simulink model "program_nova_torque_vectoring_001_2015b"  (R2016a)
settings: Solver=FixedStepAuto  StartTime=0.0  StopTime=10.0  RelTol=1e-3
PreLoadFcn:
  | dataCar
  | load_vars
  | readFuzzyFile
  | structAero
  | structEstimPar
  | structSensors
  | structSettings
PostLoadFcn:
  | , if any(exist('dsrtsu_mdlpostloadfcn', 'file') == [2, 3, 6]), try dsrtsu_mdlpostloadfcn('Execute', bdroot); catch fprintf('Error in PostLoadFcn (dsrtsu_mdlpostloadfcn) for model "%s":\n %s\n', bdroot, lasterr); end, end,
InitFcn:
  | dataCar
  | load_vars
  | readFuzzyFile
  | structAero
  | structEstimPar
  | structSensors
  | structSettings
StartFcn:
  | dataCar
  | load_vars
  | readFuzzyFile
  | structAero
  | structEstimPar
  | structSensors
  | structSettings
values from neighbouring files (symbols this model uses):
  Throttle2_offset = 500    [load_vars.m]
  Throttle_limits = [0.15, 0.90, 0.16, 0.92]    [load_vars.m]
libraries: rtican x42, hdlsllib x32, simulink x3, fuzblock x1
(part 11 of 11)

== matlab function program_nova_torque_vectoring_001_2015b/Processor/Vehicle Estimated Parameters/Fy Estimator  ==
  data: sensors input; Fyi output; settings input; Fzi input; Fxi input; car parameter
function Fyi = Fy_Estimator(sensors, settings, Fzi, Fxi, car)

Fyi=[0;0;0;0];
persistent yawRatePrev; if isempty(yawRatePrev); yawRatePrev = sensors.yawRate; end
persistent M_Fx; if isempty(M_Fx); M_Fx = 0; end
persistent M_Fy; if isempty(M_Fy); M_Fy = 0; end
persistent FyRear; if isempty(FyRear); FyRear = 0; end
persistent FzRatioFront; if isempty(FzRatioFront);FzRatioFront = 0; end
persistent FzRatioRear; if isempty(FzRatioRear); FzRatioRear = 0; end
persistent FyFront; if isempty(FyFront); FyFront = 0; end
persistent Fy_FL; if isempty(Fy_FL); Fy_FL = 0; end

scaleFactorFy = 0.7;

yawAcc = (sensors.yawRate - yawRatePrev) * car.fECU;

wheelAngle = (sensors.wheelAngles(1)+sensors.wheelAngles(2))/2;

%Calculate contributions to the moment from lateral forces through the
%total yaw moment and moment of the longitudinal forces.
M_YawTot = car.yawInertia*yawAcc;
M_Fx = (car.tw/2)*cos(wheelAngle)*(Fxi(1)-Fxi(2))...
    +car.lf*sin(wheelAngle)*(Fxi(1)+Fxi(2))...
    +(car.tw/2)*(Fxi(3)-Fxi(4));
M_Fy = M_YawTot - M_Fx;

%Distribution of lateral force on front and rear axle
%NOTE %sin(steerinAngle) deel wordt momenteel verwaarloosd
%     %--> FyFR - FyFL =~ 0
Fy = car.mass*sensors.ay;
FyRear = (cos(wheelAngle)*car.lf*Fy - M_Fy)/...
    (cos(wheelAngle)*car.lf+car.lr);
FyFront = Fy - FyRear;

%Distribution of lateral force on left and right tire by using the normal
%force distribution.

%Use of a scale factor 

FzRatioFront = [Fzi(1); Fzi(2)]./sum(Fzi(1:2));
FzRatioRear = [Fzi(3); Fzi(4)]./sum(Fzi(3:4));



FyFrontDiff = (FzRatioFront(1) - FzRatioFront(2))*scaleFactorFy/2;
Fy_FL = FyFront/2 + FyFrontDiff* FyFront;
Fy_FR = FyFront/2 - FyFrontDiff* FyFront;
FyRearDiff = (FzRatioRear(1) - FzRatioRear(2))*scaleFactorFy/2;
Fy_RL = FyRear/2 + FyRearDiff* FyRear;
Fy_RR = FyRear/2 - FyRearDiff* FyRear;
    
Fyi=[Fy_FL;Fy_FR;Fy_RL;Fy_RR];

yawRatePrev=sensors.yawRate;

== matlab function program_nova_torque_vectoring_001_2015b/Processor/Vehicle Estimated Parameters/Fz Estimator  ==
  data: sensors input; Fzi output; settings input; v input; car parameter; aero input
function Fzi = Fz_Estimator(sensors, settings, v,car, aero)
if isempty(v); v =0;end
%Dynamical loads 
%Without taking suspension into account


FFA = car.g*car.mass*car.lr/car.wb - (car.h/car.wb)*(car.mass*sensors.ax) - aero.FD*((car.h+aero.lever_FD(2))/car.wb) - aero.FL*((car.lr-aero.lever_FL(1))/car.wb); %dyn load Front Axle
FRA = car.g*car.mass*car.lf/car.wb + (car.h/car.wb)*(car.mass*sensors.ax) + aero.FD*((car.h+aero.lever_FD(2))/car.wb) - aero.FL*((car.lf+aero.lever_FL(1))/car.wb); %dyn load Rear Axle


FFL = FFA/2 - (car.h/(2*car.tw))*(car.mass*sensors.ay);
FFR = FFA/2 + (car.h/(2*car.tw))*(car.mass*sensors.ay);
FRL = FRA/2 - (car.h/(2*car.tw))*(car.mass*sensors.ay);
FRR = FRA/2 + (car.h/(2*car.tw))*(car.mass*sensors.ay);


Fzi = [FFL;FFR;FRL;FRR];

== matlab function program_nova_torque_vectoring_001_2015b/Processor/Vehicle Estimated Parameters/Mu&Slip Estimator ==
  data: sensors input; mu output; settings input; slip output; v input; car parameter
function [mu,slip]= mu_slip(sensors, settings,v,car)
if isempty(v); v =0;end
yawRate = [0;0;sensors.yawRate];
dist = [car.lf car.lf -car.lr -car.lr;
    car.tw/2 -car.tw/2 car.tw/2 -car.tw/2;
    0 0 0 0];
wheelAngle = (sensors.wheelAngles(1)+sensors.wheelAngles(2))/2;

mu=[car.mu;car.mu;car.mu;car.mu];

omegaR = sensors.wheelspeed*car.tireRadius;
vWheel=zeros(4,1);
vWheel_m=zeros(3,4);

for i=1:4;
    v_sleep=cross(yawRate,dist(:,i));
    vWheel_m(:,i) = [v;0;0] + v_sleep;
    vWheel(i,1) = sqrt(vWheel_m(1,i)^2+vWheel_m(2,i)^2);
end

%state.slipRatio = (sensor.omegaiWheel * car.wheelRadius - wvi)./max((sensor.omegaiWheel * car.wheelRadius),1);

if sensors.ax > 0
    slip = (omegaR - vWheel)./omegaR;
elseif sensors.ax < 0
    slip = (omegaR - vWheel)./vWheel;
else
    slip = [0;0;0;0];
end
end

== matlab function program_nova_torque_vectoring_001_2015b/Processor/Vehicle Estimated Parameters/Velocity Estimator/Fuzzy Velocity/FuzzyVelicityGenerator ==
  data: k1 input; vFuzzy output; k2 input; k3 input; k4 input; k5 input; sensors input; settings input; car parameter
function vFuzzy = fuzzyVelocityGenerator(k1,k2,k3,k4,k5,sensors,settings,car)

persistent vFuzzyPrev; if isempty(vFuzzyPrev); vFuzzyPrev = 0; end

beta=0;


vRFL_COG = (sensors.wheelspeed(1)*car.tireRadius...
    + sensors.yawRate*(car.tw/2-car.lf*beta))...
    *cos(sensors.wheelAngles(1)-beta);
vRFR_COG = (sensors.wheelspeed(2)*car.tireRadius...
    - sensors.yawRate*(car.tw/2+car.lf*beta))...
    *cos(sensors.wheelAngles(2)-beta);
vRRL_COG = (sensors.wheelspeed(3)*car.tireRadius...
    + sensors.yawRate*(car.tw/2+car.lr*beta))...
    *cos(beta);
vRRR_COG = (sensors.wheelspeed(4)*car.tireRadius...
    - sensors.yawRate*(car.tw/2-car.lr*beta))...
    *cos(beta);
vR_COG=[vRFL_COG;vRFR_COG;vRRL_COG;vRRR_COG];

vFuzzy = (sum([k1;k2;k3;k4].*vR_COG)+k5*(vFuzzyPrev+car.dt*sensors.ax))...
    /(k1+k2+k3+k4+k5);

vFuzzyPrev = vFuzzy;

== matlab function program_nova_torque_vectoring_001_2015b/Processor/Vehicle Estimated Parameters/Velocity Estimator/Fuzzy Velocity/fuzzyParam ==
  data: sensors input; deltaVFL output; settings input; vFuzzyPrev input; deltaVFR output; deltaVRL output; deltaVRR output; maxDeltaV output; car parameter
function [deltaVFL,deltaVFR,deltaVRL,deltaVRR,maxDeltaV]= fuzzyParam(sensors, settings,vFuzzyPrev,car)
beta=0;
vRFL_COG = (sensors.wheelspeed(1)*car.tireRadius...
    + sensors.yawRate*(car.tw/2-car.lf*beta))...
    *cos(sensors.wheelAngles(1)-beta);
vRFR_COG = (sensors.wheelspeed(2)*car.tireRadius...
    - sensors.yawRate*(car.tw/2+car.lf*beta))...
    *cos(sensors.wheelAngles(2)-beta);
vRRL_COG = (sensors.wheelspeed(3)*car.tireRadius...
    + sensors.yawRate*(car.tw/2+car.lr*beta))...
    *cos(beta);
vRRR_COG = (sensors.wheelspeed(4)*car.tireRadius...
    - sensors.yawRate*(car.tw/2-car.lr*beta))...
    *cos(beta);
vR_COG=[vRFL_COG;vRFR_COG;vRRL_COG;vRRR_COG];

deltaVFL = vRFL_COG-vFuzzyPrev;
deltaVFR = vRFR_COG-vFuzzyPrev;
deltaVRL = vRRL_COG-vFuzzyPrev;
deltaVRR = vRRR_COG-vFuzzyPrev;

maxDeltaV = abs(vFuzzyPrev-max(vR_COG))+abs(vFuzzyPrev-min(vR_COG));

== matlab function program_nova_torque_vectoring_001_2015b/Processor/Vehicle Estimated Parameters/Velocity Estimator/Kalman Velocity ==
  data: sensors input; settings input; v2 input; vKalman output; v4 input; car parameter
function vKalman = Velocity_EstimatorKalman(sensors,settings,v2,v4,car)


% Keep track of the estimated velocity
persistent vEst; if isempty(vEst); vEst = 0; end;
persistent PEst; if isempty(PEst); PEst = 0; end;

% Model
A = 1; B = car.dt;
H = [1;1];
Q = car.kalmanVelocity.Q;
R = car.kalmanVelocity.R;

% Measurements
y = [v2; v4];

% if settings.velocityEstimation == 0 || settings.velocityEstimation == 1 || vEst < car.speed.velTreshold || sensors.vboxX < car.speed.velTreshold
%     %vbox disabled
%     H(1) = 0;
% end



% === Time update ===
vEst = A*vEst + B*sensors.ax;
PEst = A*PEst*A' + Q;

% === Measurement update ===
K = PEst*H'/(H*PEst*H'+R);
vEst = vEst + K*(y-H*vEst);
PEst = (1-K*H)*PEst;
% Output
vest_out = vEst;

%sensors_out = sensors;
%sensors_out.vx = vest_out;
vKalman = vest_out;

== matlab function program_nova_torque_vectoring_001_2015b/Processor/Vehicle Estimated Parameters/Velocity Estimator/MATLAB Function ==
  data: v output; vFuzzy input
function v = fcn(vFuzzy)
%#codegen

v = vFuzzy;

== matlab function program_nova_torque_vectoring_001_2015b/Processor/Vehicle Estimated Parameters/Velocity Estimator/Velicity Estimator 2 ==
  data: sensors input; v2 output; settings input; car parameter; vCOG output
function [v2,vCOG] = Velocity_Estimator1(sensors, settings,  car)

vycog = 0;
dist = [car.lf car.lf -car.lr -car.lr;
  car.tw/2 -car.tw/2 car.tw/2 -car.tw/2;
  0 0 0 0];
wheelAngle = (sensors.wheelAngles(1)+sensors.wheelAngles(2))/2;

%tw_dist = [-car.tw/2 car.tw/2 -car.tw/2 car.tw/2];
      

% Note: axis systems X,Y,Z in car frame, x,y,z in wheel frame.
%X:forward
%Y:left
%Z:up


RxyzXYZ=[cos(wheelAngle) sin(wheelAngle) 0;
   -sin(wheelAngle) cos(wheelAngle) 0;
   0 0 1];
omega = [0 0 0 0 ;
   sensors.wheelspeed(1) sensors.wheelspeed(2) sensors.wheelspeed(3) sensors.wheelspeed(4)
   ;0 0 0 0];
radius = [0;0;-car.tireRadius];
yawRate = [0;0;sensors.yawRate];

% wheelspeed = [sensors.wheelspeed(1) sensors.wheelspeed(2) sensors.wheelspeed(3) sensors.wheelspeed(4)];
% steeringAngle = [wheelAngle;wheelAngle;0;0];
% omegaR = [sensors.wheelspeed(1); sensors.wheelspeed(2); sensors.wheelspeed(3); sensors.wheelspeed(4)].*car.tireRadius;


% persistent vCOG_m
% if isempty(vCOG_m); vCOG_m = zeros(3,4); end

% persistent vxCOG
% if isempty(vxCOG); vxCOG = zeros(4,1); end
vCOG_m = zeros(3,4);
vCOG = zeros(4,1);

%vxCOG_m = zeros(4,1);


%Can be faster without the matrices
%Slip can be taken into account by v_wheel(now=0,changing it to velocity with slip) =
%RxyzXYZ*cross(wheelspeed,tireRadius)+cross(yawRate,dist)+vXYZ
 
for i=1:4
    vCOG_m(:,i) = -(RxyzXYZ*cross(omega(:,i),radius)+cross(yawRate,dist(:,i)));  %%SteeringAngle is not yet changed for the rear wheels w
    vCOG(i,1) = sqrt(vCOG_m(1,i)^2+vCOG_m(2,i)^2);
    %vxCOG_m(i,1)=vCOG_m(1,i);
    %vxCOG(i,1)=-(cos(steeringAngle(i))*(car.tireRadius*wheelspeed(i))-sensors.yawRate*tw_dist(i));
end

% Select/average based on wheel speed
axtol = 2; % Tolerance to detect acceleration / deceleration [m/s2]
if sensors.ax > axtol
    vEst_wheels = min(vCOG);    %lowest wheelspeed to take possible slip into account
elseif sensors.ax < -axtol
    vEst_wheels = max(vCOG);    %highest wheelspeed to take possible wheel lock into account
else
    vEst_wheels = median(vCOG); % Note: median is less sensitive to outliers
end




v2= vEst_wheels;

== matlab function program_nova_torque_vectoring_001_2015b/Processor/Vehicle Estimated Parameters/Velocity Estimator/Velocity Estimator 1 ==
  data: sensors input; v1 output; settings input; car parameter
function v1  = Velocity_Estimator1(sensors, settings,  car)

%x-axis forward
%y-axis left
%z-axis upwards

tw_dist = [car.tw/2; -car.tw/2; car.tw/2; -car.tw/2];    

omegaR = max(sensors.wheelspeed*car.tireRadius,0);

persistent v_last; if (isempty(v_last)); v_last = 0; end

%estimate vi
vi = omegaR - tw_dist.*sensors.yawRate;
vi = vi .* cos(sensors.wheelAngles); 

%Front/rear best speed estimation
ax=sensors.ax;
limitax = 10;

vl = vi([1 3]);
vr = vi([2 4]);

if (ax > limitax)
   vsetl=min(vl);
   vsetr=min(vr);
elseif (ax < -limitax)
   vsetl=max(vl);
   vsetr=max(vr);
else
   vsetl=(min(vl)*(limitax + ax) + max(vl)*(limitax - ax))/(2*limitax);
   vsetr=(min(vr)*(limitax + ax) + max(vr)*(limitax - ax))/(2*limitax);
end
    
%left/right best speed estimation
ay=sensors.ay;
limitay = 20;

if (ay > limitay)
   v_est = vsetr;
elseif (ay < -limitay)
   v_est = vsetl;
else
   v_est = (vsetr*(ay + limitay) + vsetl*(limitay-ay))/(2*limitay);
end

v1=v_est;
%v=mean(omegaR);

== matlab function program_nova_torque_vectoring_001_2015b/Processor/Vehicle Estimated Parameters/Velocity Estimator/Velocity_Estimator3 ==
  data: sensors input; v3 output; settings input; car parameter; v input
function v3  = Velocity_Estimator3(sensors, settings,  car, v)

persistent vActual; if isempty(vActual); vActual = 0; end


%IMPORTANT: change car.fECU and car.dt when changing operating speed in Simulink

v3 = vActual + sensors.ax * car.dt;

vActual = v;

== matlab function program_nova_torque_vectoring_001_2015b/Processor/Vehicle Estimated Parameters/Velocity Estimator/Velocity_Estimator4 ==
  data: sensors input; v4 output; settings input; Fyi input; car parameter
function v4  = Velocity_Estimator4(sensors, settings,Fyi,  car)

% Based on "Vehicle velocity estimation using effective inertia for an in-wheel
% elecric vehicle"

SumLongitudinalForce=0;




persistent wheelspeedPrev; if isempty(wheelspeedPrev); wheelspeedPrev = [0 ;0 ;0 ;0]; end
persistent vPrev; if isempty(vPrev); vPrev = 0; end
persistent v4dot; if isempty(v4dot); v4dot = 0; end
wheelspeed = sensors.wheelspeed;

alpha = (wheelspeed - wheelspeedPrev)/car.dt;

Fresist = 0.5*car.Cd*car.AFront*car.rhoAir*vPrev^2; % moet nauwkeuriger


SumLongitudinalForce = sum(sensors.torque-alpha*car.tireInertia)/car.tireRadius...
    - Fresist;
Meff = SumLongitudinalForce/sensors.ax; %effective inertia / virtual mass


v4dot = (-(Fyi(1)*sin(sensors.wheelAngles(1))+Fyi(2)*sin(sensors.wheelAngles(2)))...
    + SumLongitudinalForce) / Meff;




v4 = vPrev + v4dot*car.dt;

vPrev = v4;




end

== matlab function program_nova_torque_vectoring_001_2015b/Processor/Vehicle Estimated Parameters/Yaw Rate Reference ==
  data: sensors input; rref output; settings input; v input; car parameter
function rref = yawRateRef(sensors, settings, v, car)
if isempty(v); v =0;end
%Ackermann
wheelAngle = (sensors.wheelAngles(1)+sensors.wheelAngles(2))/2;
rref = wheelAngle*v/car.wb;




% 
% des_yaw_rate = vx*steering_angle / ...
%     (L_f + L_r + ...
%     m_chassis*vx^2*(L_r*(C_x_alpha_RL+C_x_alpha_RR)-L_f*(C_x_alpha_FL+C_x_alpha_FR))/...
%     ((C_x_alpha_RL+C_x_alpha_RR)*(C_x_alpha_FL+C_x_alpha_FR)*L));

== matlab function program_nova_torque_vectoring_001_2015b/Processor/Sensors ==
  data: ax input; sensors output Bus: sensorBus size=1; ay input; yawRate input; steeringAngle input; steerAngleFL input; steerAngleFR input; throttle input; brake input; wheelspeed_FL input; wheelspeed_FR input; wheelspeed_RL input; wheelspeed_RR input; torqueFL input; torqueFR input; torqueRL input; torqueRR input; P_elec input
function sensors = sensors(ax,ay,yawRate,steeringAngle,steerAngleFL,steerAngleFR, throttle,brake,wheelspeed_FL,wheelspeed_FR,wheelspeed_RL,wheelspeed_RR,torqueFL,torqueFR,torqueRL,torqueRR,P_elec)

sensors.ax = ax;
if ax > 50 || ax < -50
    sensors.ax_error = 1;
else
    sensors.ax_error = 0;
end
sensors.ay = ay;
if ay > 50 || ay < -50
    sensors.ay_error = 1;
else
    sensors.ay_error = 0;
end

sensors.wheelspeed = [wheelspeed_FL;wheelspeed_FR;wheelspeed_RL;wheelspeed_RR];
if wheelspeed_FL > 20000 || wheelspeed_FL < -1000
    sensors.wheelspeed_error = 1;
elseif wheelspeed_FR > 20000 || wheelspeed_FR < -1000
    sensors.wheelspeed_error = 1;
elseif wheelspeed_RL > 20000 || wheelspeed_RL < -1000
    sensors.wheelspeed_error = 1;
elseif wheelspeed_RR > 20000 || wheelspeed_RR < -1000
    sensors.wheelspeed_error = 1;
else
    sensors.wheelspeed_error = 0;
end
sensors.wheelspeed = sensors.wheelspeed./60.*2.*pi; %rpm to rad/s

sensors.yawRate = yawRate;
if yawRate > 50 || yawRate < -50
    sensors.yawRate_error = 1;
else
    sensors.yawRate_error = 0;
end

sensors.steerAngle = steeringAngle;
if steerAngle > 300 || steerAngle < -300
    sensors.steerAngle_error = 1;
else
    sensors.steerAngle_error = 0;
end

sensors.wheelAngles = [steerAngleFL;steerAngleFR;0;0];
if wheelAngles(1) > 40 || wheelAngles(1) < -40
    sensors.wheelAngle_error = 1;
elseif wheelAngles(2) > 40 || wheelAngles(2) < -40
    sensors.wheelAngle_error = 1;
else
    sensors.wheelAngle_error = 0;
end

sensors.throttle = throttle;
if throttle > 100 || throttle < 0
    sensors.throttle_error = 1;
else
    sensors.throttle_error = 0;
end
sensors.brake= brake;
if brake > 100 || brake < 0
    sensors.brake_error = 1;
else
    sensors.brake_error = 0;
end

sensors.torque = [torqueFL;torqueFR;torqueRL;torqueRR];
if torqueFL > 25 || torqueFL < -25
    sensors.torque_error = 1;
elseif torqueFR > 25 || torqueFR < -25
    sensors.torque_error = 1;
elseif torqueRL > 25 || torqueRL < -25
    sensors.torque_error = 1;
elseif torqueRR > 25 || torqueRR < -25
    sensors.torque_error = 1;
else
    sensors.torque_error = 0;
end

sensors.P_elec = P_elec;
if P_elec > 160 || P_elec_FL < 0
    sensors.P_elec_error = 1;
else
    sensors.P_elec_error = 0;
end

sensors.errors = [sensors.ax_error;sensors.ay_error;sensors.wheelspeed_error;...
    sensors.yawRate_error;sensors.wheelAngle_error;throttle_error,brake_error;...
    sensors.torque_error;sensors.P_elec_error];
sensors.TCRE = [sensors.ax_error;sensors.ay_error;sensors.wheelspeed_error;...
    throttle_error,brake_error;sensors.torque_error;sensors.P_elec_error];
    %Traction Control Relevant Errors

== matlab function program_nova_torque_vectoring_001_2015b/Processor/Ackermann Arno ==
  data: x input; thetaL output; thetaR output
function [thetaL, thetaR]= ackerman(x)
%x is de rack travel in mm
%+ als rack naar rechts beweegt van achter de wagen bekeken
%- als rack naar links beweegt van achter de wagen bekeken

thetaL=-2*(10^-9)*(x^6)+8*(10^-8)*(x^5)+9*(10^-7)*(x^4)+3*(10^-5)*(x^3)-0.0049*(x^2)+1.0437*x+0.0254;
%thetaL is hoeverdraaiing van linker wiel in °
%-hoek is draaien naar links van boven de wagen bekeken
%+hoek is draaien naar rechts van boven de wagen bekeken

thetaR=2*(10^-9)*(x^6)+8*(10^-8)*(x^5)-9*(10^-7)*(x^4)+3*(10^-5)*(x^3)+0.0049*(x^2)+1.0437*x-0.0254;
%thetaR is hoekverdraaiing van rechter wiel in °
%-hoek is draaien naar links van boven de wagen bekeken
%+hoek is draaien naar rechts van boven de wagen bekeken

end
